simulink model "MBD_W1_P1"  (R2020a)
settings: Solver=VariableStepAuto  StartTime=0.0  StopTime=Te  MaxStep=0.001  RelTol=1e-3
values from neighbouring files (symbols this model uses):
  b = 50    [MBD_W1_P1_init.m]
  K1 = 50    [MBD_W1_P1_init.m]
  K12 = 1.6    [MBD_W1_P1_init.m]
  M1 = 100    [MBD_W1_P1_init.m]
  M2 = 30    [MBD_W1_P1_init.m]
settings Model: Creator=Atri Mondal  LastModifiedBy=Atri Mondal

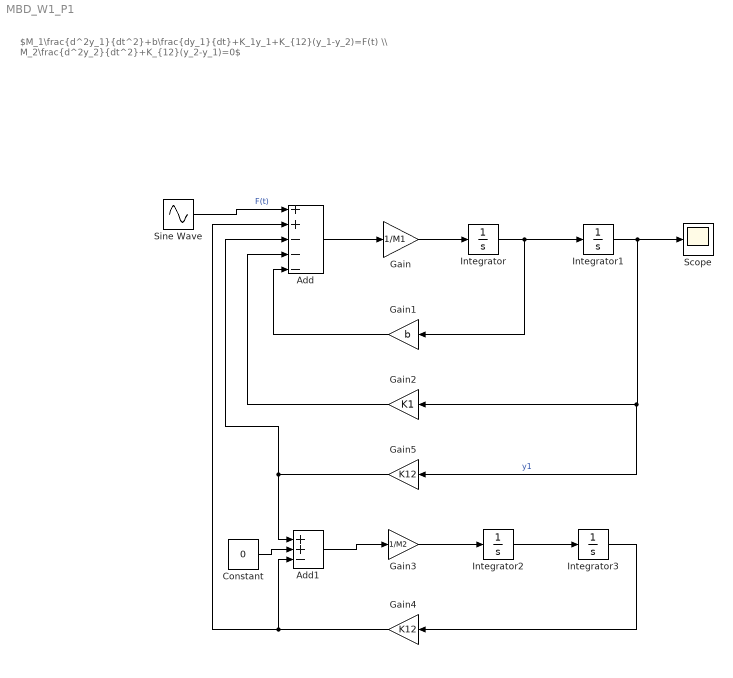
== system MBD_W1_P1 ==
  note: $M_1\frac{d^2y_1}{dt^2}+b\frac{dy_1}{dt}+K_1y_1+K_{12}(y_1-y_2)=F(t) \\ M_2\frac{d^2y_2}{dt^2}+K_{12}(y_2-y_1)=0$
  Add : Sum  Inputs=++---
  Add1 : Sum  Inputs=++-
  Constant : Constant  Value=0
  Gain : Gain  Gain=1/M1
  Gain1 : Gain  Gain=b
  Gain2 : Gain  Gain=K1
  Gain3 : Gain  Gain=1/M2
  Gain4 : Gain  Gain=K12
  Gain5 : Gain  Gain=K12
  Integrator{,1..3} (4 alike) : Integrator
  Scope : Scope
  Sine Wave : Sin  Amplitude=2  Frequency=10  SampleTime=0
  wires:
  Constant/1 -> Add1/2
  Integrator3/1 -> Gain4/1
  Gain2/1 -> Add/4
  Gain5/1 -> Add1/1, Add/3
  Gain1/1 -> Add/5
  Gain3/1 -> Integrator2/1
  Gain4/1 -> Add1/3, Add/2
  Integrator2/1 -> Integrator3/1
  Integrator1/1 -> Scope/1, Gain5/1, Gain2/1  "y1"
  Add1/1 -> Gain3/1
  Integrator/1 -> Gain1/1, Integrator1/1
  Gain/1 -> Integrator/1
  Add/1 -> Gain/1
  Sine Wave/1 -> Add/1  "F(t)"
